simulink model "sim_trot"  (R2025b)
settings: Solver=VariableStepAuto  StartTime=0.0  StopTime=t_sim  RelTol=1e-3
undefined symbols (not defined in the file): C14, C2, C5, K, Kh, Ki, L, R, R5, R6, R7, Si
settings Model: Creator=thibaut  LastModifiedBy=thibaut

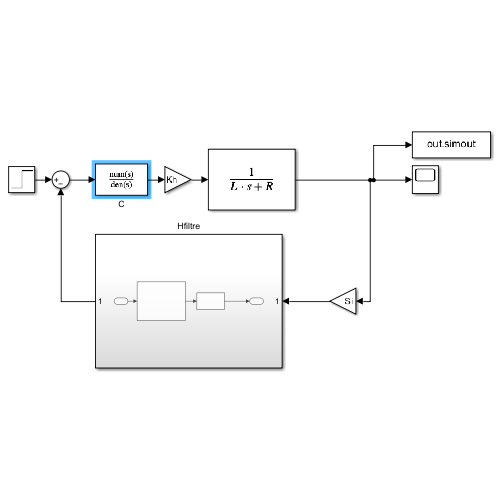
[thumbnail: Simulink's stored preview of the top-level diagram]
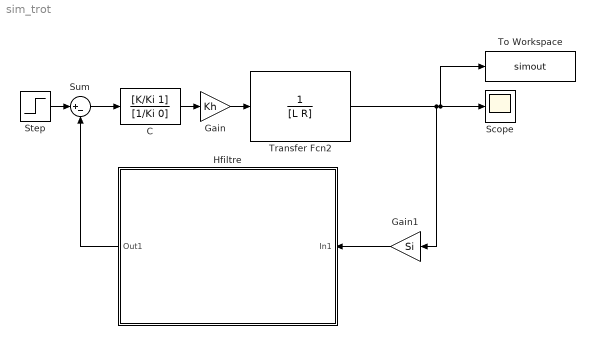
== system sim_trot ==
  C : TransferFcn  Numerator=[K/Ki 1]  Denominator=[1/Ki 0]
  Gain : Gain  Gain=Kh
  Gain1 : Gain  Gain=Si
  Hfiltre : Subsystem
  Scope : Scope
      settings: ActiveDisplayYMinimum=-1  ActiveDisplayYMaximum=1
  Step : Step  Time=0  SampleTime=0
  Sum : Sum  Inputs=|+-
  To Workspace : ToWorkspace  VariableName=simout  SaveFormat=Timeseries  SampleTime=-1
  Transfer Fcn2 : TransferFcn  Denominator=[L R]
  wires:
  Sum/1 -> C/1
  C/1 -> Gain/1
  Gain/1 -> Transfer Fcn2/1
  Transfer Fcn2/1 -> To Workspace/1, Scope/1, Gain1/1
  Gain1/1 -> Hfiltre/1(In1)
  Hfiltre/1(Out1) -> Sum/2
  Step/1 -> Sum/1

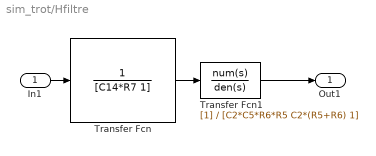
== system sim_trot/Hfiltre ==
  In1 : Inport
  Transfer Fcn : TransferFcn  Denominator=[C14*R7 1]
  Transfer Fcn1 : TransferFcn  Denominator=[C2*C5*R6*R5 C2*(R5+R6) 1]
  Out1 : Outport
  wires:
  In1/1 -> Transfer Fcn/1
  Transfer Fcn/1 -> Transfer Fcn1/1
  Transfer Fcn1/1 -> Out1/1
